simulink model "EngineModel_scaled_27_7_2016_with_new_maps"  (R2021a)
settings: Solver=ode4  StartTime=0.0  StopTime=30  FixedStep=0.2  RelTol=1e-3  EnableMultiTasking=on
values from neighbouring files (symbols this model uses):
  Fanmap_2 = [1 1 1 1 1 1 1 1 1 1 275.724 325.4224 ... (330 elements, 10x3x11)]    [enginemaps2.mat]
  HPCompmap_2 = [1 1 1 1 1 1 1 1 1 1 32.390865 37.6623195 ... (330 elements, 10x3x11)]    [enginemaps2.mat]
  HPTurbinemap_2 = [0.24979968 0.24979968 0.24979968 0.24979968 0.24979968 0.24979968 0.24979968 0.24979968 0.24979968 0.24979968 0.004250667 0.005047667 ... (330 elements, 10x3x11)]    [enginemaps2.mat]
  LPCompmap_2 = [1 1 1 1 1 1 1 1 1 1 34.17260994 40.23277722 ... (330 elements, 10x3x11)]    [enginemaps2.mat]
  LPTurbinemap_2 = [0.665969797 0.665969797 0.665969797 0.665969797 0.665969797 0.665969797 0.665969797 0.665969797 0.00912 0.013173333 0.015706667 0.01672 ... (264 elements, 8x3x11)]    [enginemaps2.mat]
undefined symbols (not defined in the file or in its folder): Adiabatic_compression_fan, Adiabatic_compression_HPC, Adiabatic_compression_LPC, coldnozzle, compression_ram, cond_f2, D, datatables, hotnozzle, HPT1, if_Nth, if_Ntl, if_Z, LPT, performance1, thermo_combustor, turbo
libraries: dspmtrx3 x10, aerolibatmos2 x8, dspsigattribs x3, dspsolvers x2, dspfactors x1
(part 11 of 14)

== system EngineModel_scaled_27_7_2016_with_new_maps/Double spool TFE CF6-50 steady state modeling (BOING 747-200)/Error Due to Vs/Error Due To Dv4/HPC/HPC Map/HPComp Map Lookup Table pressure ratio ==
  Corr Speed Nch : Inport
  zch : Inport  Port=2
  3D HPC map Lookup Table pressure ratio : Lookup_n-D  NumberOfTableDimensions=3  BreakpointsForDimension1=[0.562,0.674,0.787,0.899,1,1.034,1.067,1.124,1.236,1.292]  BreakpointsForDimension2=[1,2,3]  BreakpointsForDimension3=[0,0.1,0.2,0.3,0.4,0.5,0.6,0.7,0.8,0.9,1]  IndexSearchMethod=Linear search  Table=HPCompmap_2  InterpMethod=Cubic spline  ExtrapMethod=Cubic spline  OutDataTypeStr=double  RndMeth=Simplest
      settings: InputPortMap=u0,u1,u2
  Constant1 : Constant
  Display : Display
  HPC Prch : Outport
  wires:
  Constant1/1 -> 3D HPC map Lookup Table pressure ratio/2
  Corr Speed Nch/1 -> 3D HPC map Lookup Table pressure ratio/1
  3D HPC map Lookup Table pressure ratio/1 -> HPC Prch/1, Display/1
  zch/1 -> 3D HPC map Lookup Table pressure ratio/3

== system EngineModel_scaled_27_7_2016_with_new_maps/Double spool TFE CF6-50 steady state modeling (BOING 747-200)/Error Due to Vs/Error Due To Dv4/HPC/HPC Map/If condition Zch ==
  Zchi : Inport
  Demux : Demux  Outputs=1
      settings: DisplayOption=none
  Interpreted MATLAB Function : MATLABFcn  MATLABFcn=if_Z(u(1))  OutputDimensions=1
  Mux : Mux  Inputs=1
      settings: DisplayOption=signals
  Zch : Outport
  wires:
  Zchi/1 -> Mux/1
  Demux/1 -> Zch/1
  Mux/1 -> Interpreted MATLAB Function/1
  Interpreted MATLAB Function/1 -> Demux/1

== system EngineModel_scaled_27_7_2016_with_new_maps/Double spool TFE CF6-50 steady state modeling (BOING 747-200)/Error Due to Vs/Error Due To Dv4/HPT/enthalpy_MAPS/HPT map ==
  Nth : Inport
  TFth : Inport  Port=2
  HPT Map lookup Table (DH/T) : Subsystem
  HPT Map lookup Table Efficency : Subsystem
  (DH/T)th : Outport
  etath : Outport  Port=2
  wires:
  HPT Map lookup Table Efficency/1(HPT Ettath) -> etath/1
  HPT Map lookup Table (DH/T)/1(HPT (DH/T)th) -> (DH/T)th/1
  TFth/1 -> HPT Map lookup Table (DH/T)/2(TFth), HPT Map lookup Table Efficency/2(TFth)
  Nth/1 -> HPT Map lookup Table (DH/T)/1(corr speed Nth), HPT Map lookup Table Efficency/1(corr speed Nth)

== system EngineModel_scaled_27_7_2016_with_new_maps/Double spool TFE CF6-50 steady state modeling (BOING 747-200)/Error Due to Vs/Error Due To Dv4/HPT/enthalpy_MAPS/Nch_Nth ==
  Tt4 : Inport
  Tt2.5 : Inport  Port=2
  Nch : Inport  Port=3
  (To)Ref : Constant  Value=288
  (theta4)d : Constant  Value=1.1018
  Display5 : Display
  Product3 : Product  Inputs=***  SaturateOnIntegerOverflow=on  OutDataTypeStr=Inherit: Same as first input
  Product4 : Product  Inputs=*/  SaturateOnIntegerOverflow=on  OutDataTypeStr=Inherit: Same as first input
  Product6 : Product  Inputs=*/  SaturateOnIntegerOverflow=on  OutDataTypeStr=Inherit: Same as first input
  Product7 : Product  Inputs=*/  SaturateOnIntegerOverflow=on  OutDataTypeStr=Inherit: Same as first input
  Sqrt1 : Sqrt  SaturateOnIntegerOverflow=on
  Sqrt2 : Sqrt  SaturateOnIntegerOverflow=on
  const. : Constant  Value=100
  Nth : Outport
  wires:
  Nch/1 -> Product3/3
  Sqrt2/1 -> Product6/1
  Product6/1 -> Product3/2
  (theta4)d/1 -> Product6/2
  Product4/1 -> Sqrt2/1
  Tt2.5/1 -> Product4/1
  Tt4/1 -> Sqrt1/1
  Product3/1 -> Display5/1, Nth/1
  const./1 -> Product7/1
  Sqrt1/1 -> Product7/2
  (To)Ref/1 -> Product4/2
  Product7/1 -> Product3/1

== system EngineModel_scaled_27_7_2016_with_new_maps/Double spool TFE CF6-50 steady state modeling (BOING 747-200)/Error Due to Vs/Error Due To Dv4/LPC/Adiabatic compression/isentropic compression ==
  Tt13 : Inport
  Prcl : Inport  Port=2
  P13 : Inport  Port=3
  Ht13 : Inport  Port=4
  S13 : Inport  Port=5
  etacl : Inport  Port=6
  Demux : Demux
      settings: DisplayOption=none
  Interpreted MATLAB Function : MATLABFcn  MATLABFcn=Adiabatic_compression_LPC(u(1),u(2),u(3),u(4),u(5),u(6))  OutputDimensions=4
  Mux : Mux  Inputs=6
      settings: DisplayOption=signals
  S25 : Outport
  Tt25 : Outport  Port=2
  Pt25 : Outport  Port=3
  Ht25 : Outport  Port=4
  wires:
  Demux/4 -> Ht25/1
  etacl/1 -> Mux/6
  Demux/3 -> S25/1
  S13/1 -> Mux/5
  Ht13/1 -> Mux/4
  Prcl/1 -> Mux/2
  P13/1 -> Mux/3
  Mux/1 -> Interpreted MATLAB Function/1
  Demux/1 -> Tt25/1
  Interpreted MATLAB Function/1 -> Demux/1
  Demux/2 -> Pt25/1
  Tt13/1 -> Mux/1

== system EngineModel_scaled_27_7_2016_with_new_maps/Double spool TFE CF6-50 steady state modeling (BOING 747-200)/Error Due to Vs/Error Due To Dv4/LPC/LPC Map/If condition Zcl ==
  Zcli : Inport
  Demux : Demux  Outputs=1
      settings: DisplayOption=none
  Interpreted MATLAB Function : MATLABFcn  MATLABFcn=if_Z(u(1))  OutputDimensions=1
  Mux : Mux  Inputs=1
      settings: DisplayOption=signals
  Zcl : Outport
  wires:
  Zcli/1 -> Mux/1
  Demux/1 -> Zcl/1
  Mux/1 -> Interpreted MATLAB Function/1
  Interpreted MATLAB Function/1 -> Demux/1

== system EngineModel_scaled_27_7_2016_with_new_maps/Double spool TFE CF6-50 steady state modeling (BOING 747-200)/Error Due to Vs/Error Due To Dv4/LPC/LPC Map/LPC Map Lookuptable efficiency ==
  corr Speed Ncl : Inport
  Zcl : Inport  Port=2
  3D fanmap Lookup Table : Lookup_n-D  NumberOfTableDimensions=3  BreakpointsForDimension1=[0.3,0.4,0.5,0.6,0.7,0.8,0.9,1.0,1.1,1.2]  BreakpointsForDimension2=[1,2,3]  BreakpointsForDimension3=[0,0.1,0.2,0.3,0.4,0.5,0.6,0.7,0.8,0.9,1]  IndexSearchMethod=Linear search  Table=LPCompmap_2  InterpMethod=Cubic spline  ExtrapMethod=Cubic spline  OutDataTypeStr=double  RndMeth=Simplest
      settings: InputPortMap=u0,u1,u2
  Constant1 : Constant  Value=3
  Display : Display
  etacl : Outport
  wires:
  Zcl/1 -> 3D fanmap Lookup Table/3
  3D fanmap Lookup Table/1 -> Display/1, etacl/1
  Constant1/1 -> 3D fanmap Lookup Table/2
  corr Speed Ncl/1 -> 3D fanmap Lookup Table/1

== system EngineModel_scaled_27_7_2016_with_new_maps/Double spool TFE CF6-50 steady state modeling (BOING 747-200)/Error Due to Vs/Error Due To Dv4/LPC/LPC Map/LPC Map Lookuptable massflow ==
  corr Speed Ncl : Inport
  Zcl : Inport  Port=2
  3D fanmap Lookup Table : Lookup_n-D  NumberOfTableDimensions=3  BreakpointsForDimension1=[0.3,0.4,0.5,0.6,0.7,0.8,0.9,1.0,1.1,1.2]  BreakpointsForDimension2=[1,2,3]  BreakpointsForDimension3=[0,0.1,0.2,0.3,0.4,0.5,0.6,0.7,0.8,0.9,1]  IndexSearchMethod=Linear search  Table=LPCompmap_2  InterpMethod=Cubic spline  ExtrapMethod=Cubic spline  OutDataTypeStr=double  RndMeth=Simplest
      settings: InputPortMap=u0,u1,u2
  Constant1 : Constant  Value=2
  Display : Display
  " MFPcl" : Outport
  wires:
  Zcl/1 -> 3D fanmap Lookup Table/3
  3D fanmap Lookup Table/1 -> Display/1, " MFPcl"/1
  Constant1/1 -> 3D fanmap Lookup Table/2
  corr Speed Ncl/1 -> 3D fanmap Lookup Table/1

== system EngineModel_scaled_27_7_2016_with_new_maps/Double spool TFE CF6-50 steady state modeling (BOING 747-200)/Error Due to Vs/Error Due To Dv4/LPC/LPC Map/LPC Map Lookuptable pressure ratio ==
  corr Speed Ncl : Inport
  Zcl : Inport  Port=2
  3D fanmap Lookup Table : Lookup_n-D  NumberOfTableDimensions=3  BreakpointsForDimension1=[0.3,0.4,0.5,0.6,0.7,0.8,0.9,1.0,1.1,1.2]  BreakpointsForDimension2=[1,2,3]  BreakpointsForDimension3=[0,0.1,0.2,0.3,0.4,0.5,0.6,0.7,0.8,0.9,1]  IndexSearchMethod=Linear search  Table=LPCompmap_2  InterpMethod=Cubic spline  ExtrapMethod=Cubic spline  OutDataTypeStr=double  RndMeth=Simplest
      settings: InputPortMap=u0,u1,u2
  Constant1 : Constant
  Display : Display
  " Prcl" : Outport
  wires:
  corr Speed Ncl/1 -> 3D fanmap Lookup Table/1
  Constant1/1 -> 3D fanmap Lookup Table/2
  3D fanmap Lookup Table/1 -> " Prcl"/1, Display/1
  Zcl/1 -> 3D fanmap Lookup Table/3

== system EngineModel_scaled_27_7_2016_with_new_maps/Double spool TFE CF6-50 steady state modeling (BOING 747-200)/Error Due to Vs/Error Due To Dv4/LPT/enthalpy_MAPS/LPT map ==
  Ntl : Inport
  TFtl : Inport  Port=2
  LPT Map lookup Table (DH/T) : Subsystem
  LPT Map lookup Table Efficency : Subsystem
  (DH/T)tl : Outport
  etatl : Outport  Port=2
  wires:
  LPT Map lookup Table Efficency/1(HPT Ettatl) -> etatl/1
  LPT Map lookup Table (DH/T)/1(LPT (DH/T)tl) -> (DH/T)tl/1
  TFtl/1 -> LPT Map lookup Table (DH/T)/2(TFtl), LPT Map lookup Table Efficency/2(TFtl)
  Ntl/1 -> LPT Map lookup Table (DH/T)/1(corr speed Ntl), LPT Map lookup Table Efficency/1(corr speed Ntl)

== system EngineModel_scaled_27_7_2016_with_new_maps/Double spool TFE CF6-50 steady state modeling (BOING 747-200)/Error Due to Vs/Error Due To Dv4/LPT/enthalpy_MAPS/Nch_Nth ==
  Tt45 : Inport
  Tt2 : Inport  Port=2
  Ncf : Inport  Port=3
  (To)Ref : Constant  Value=288
  (theta2)d : Constant  Value=0.9532186
  Display5 : Display
  Product3 : Product  Inputs=**  SaturateOnIntegerOverflow=on  OutDataTypeStr=Inherit: Same as first input
  Product4 : Product  Inputs=*/  SaturateOnIntegerOverflow=on  OutDataTypeStr=Inherit: Same as first input
  Product6 : Product  Inputs=*/  SaturateOnIntegerOverflow=on  OutDataTypeStr=Inherit: Same as first input
  Product7 : Product  Inputs=*/  SaturateOnIntegerOverflow=on  OutDataTypeStr=Inherit: Same as first input
  Product8 : Product  Inputs=**  SaturateOnIntegerOverflow=on  OutDataTypeStr=Inherit: Same as first input
  Sqrt1 : Sqrt  SaturateOnIntegerOverflow=on
  Sqrt2 : Sqrt  SaturateOnIntegerOverflow=on
  const. : Constant  Value=100
  Ntl : Outport
  wires:
  Sqrt2/1 -> Product6/1
  Product6/1 -> Product8/2
  (theta2)d/1 -> Product6/2
  Product4/1 -> Sqrt2/1
  Tt2/1 -> Product4/1
  Tt45/1 -> Sqrt1/1
  Ncf/1 -> Product3/2
  Product3/1 -> Ntl/1, Display5/1
  const./1 -> Product7/1
  Sqrt1/1 -> Product7/2
  Product7/1 -> Product8/1
  (To)Ref/1 -> Product4/2
  Product8/1 -> Product3/1

== system EngineModel_scaled_27_7_2016_with_new_maps/Double spool TFE CF6-50 steady state modeling (BOING 747-200)/Error Due to Vs/Error Due To Dv4/Ram/If condition PRF/If Action Subsystem ==
  In1 : Inport
  Action Port : ActionPort  ActionPortLabel=if(u1 <1)
  Out1 : Outport
  wires:
  In1/1 -> Out1/1

== system EngineModel_scaled_27_7_2016_with_new_maps/Double spool TFE CF6-50 steady state modeling (BOING 747-200)/Error Due to Vs/Error Due To Dv4/Ram/If condition PRF/If Action Subsystem1 ==
  In1 : Inport
  Action Port : ActionPort  ActionPortLabel=else
  Out1 : Outport
  wires:
  In1/1 -> Out1/1

== system EngineModel_scaled_27_7_2016_with_new_maps/Double spool TFE CF6-50 steady state modeling (BOING 747-200)/Error Due to Vs/Error Due To Dv4/Ram/If condition PRF/If Action Subsystem2 ==
  In1 : Inport
  Action Port : ActionPort  ActionPortLabel=elseif(u1>5)
  Out1 : Outport
  wires:
  In1/1 -> Out1/1

== system EngineModel_scaled_27_7_2016_with_new_maps/Double spool TFE CF6-50 steady state modeling (BOING 747-200)/Error Due to Vs/Error Due To Dv5/Combustor/Thermo_combustor/Combustor thermo ==
  Pt4 : Inport
  Ht4 : Inport  Port=2
  F/A : Inport  Port=3
  Cp3 : Inport  Port=4
  Demux : Demux
      settings: DisplayOption=none
  Interpreted MATLAB Function : MATLABFcn  MATLABFcn=thermo_combustor(u(1),u(2),u(3),u(4))  OutputDimensions=4
  Mux : Mux
      settings: DisplayOption=signals
  Tt4 : Outport
  S4 : Outport  Port=2
  Cp4 : Outport  Port=3
  Mw4 : Outport  Port=4
  wires:
  Mux/1 -> Interpreted MATLAB Function/1
  Interpreted MATLAB Function/1 -> Demux/1
  Ht4/1 -> Mux/2
  Pt4/1 -> Mux/1
  F/A/1 -> Mux/3
  Demux/1 -> Tt4/1
  Demux/2 -> S4/1
  Demux/3 -> Cp4/1
  Demux/4 -> Mw4/1
  Cp3/1 -> Mux/4

== system EngineModel_scaled_27_7_2016_with_new_maps/Double spool TFE CF6-50 steady state modeling (BOING 747-200)/Error Due to Vs/Error Due To Dv5/Combustor/combustor o//p pressure/If Action Subsystem ==
  In1 : Inport
  Action Port : ActionPort  ActionPortLabel=if(u1 > 1)
  Out1 : Outport
  wires:
  In1/1 -> Out1/1

== system EngineModel_scaled_27_7_2016_with_new_maps/Double spool TFE CF6-50 steady state modeling (BOING 747-200)/Error Due to Vs/Error Due To Dv5/Combustor/combustor o//p pressure/If Action Subsystem1 ==
  In1 : Inport
  Action Port : ActionPort  ActionPortLabel=else
  Out1 : Outport
  wires:
  In1/1 -> Out1/1

== system EngineModel_scaled_27_7_2016_with_new_maps/Double spool TFE CF6-50 steady state modeling (BOING 747-200)/Error Due to Vs/Error Due To Dv5/Fan/Adiabatic compression/isentropic compression ==
  Tt2 : Inport
  Pr : Inport  Port=2
  Pt2 : Inport  Port=3
  Ht2 : Inport  Port=4
  S2 : Inport  Port=5
  etaf : Inport  Port=6
  Demux : Demux
      settings: DisplayOption=none
  Interpreted MATLAB Function : MATLABFcn  MATLABFcn=Adiabatic_compression_fan(u(1),u(2),u(3),u(4),u(5),u(6))  OutputDimensions=4
  Mux : Mux  Inputs=6
      settings: DisplayOption=signals
  S13 : Outport
  Tt13 : Outport  Port=2
  Pt13 : Outport  Port=3
  Ht13 : Outport  Port=4
  wires:
  Tt2/1 -> Mux/1
  Demux/2 -> Pt13/1
  Interpreted MATLAB Function/1 -> Demux/1
  Demux/1 -> Tt13/1
  Mux/1 -> Interpreted MATLAB Function/1
  Pt2/1 -> Mux/3
  Pr/1 -> Mux/2
  Ht2/1 -> Mux/4
  S2/1 -> Mux/5
  Demux/3 -> S13/1
  etaf/1 -> Mux/6
  Demux/4 -> Ht13/1

== system EngineModel_scaled_27_7_2016_with_new_maps/Double spool TFE CF6-50 steady state modeling (BOING 747-200)/Error Due to Vs/Error Due To Dv5/Fan/Fan Map/Fan Map Lookuptable mass flow ==
  Ncf : Inport
  Zf : Inport  Port=2
  Constant : Constant  Value=2
  Display : Display
  massflow 3D fanmap Lookup Table : Lookup_n-D  NumberOfTableDimensions=3  BreakpointsForDimension1=[0.3,0.4,0.5,0.6,0.7,0.8,0.9,1.0,1.1,1.2]  BreakpointsForDimension2=[1,2,3]  BreakpointsForDimension3=[0,0.1,0.2,0.3,0.4,0.5,0.6,0.7,0.8,0.9,1]  IndexSearchMethod=Linear search  Table=Fanmap_2  InterpMethod=Cubic spline  ExtrapMethod=Cubic spline  OutDataTypeStr=double  RndMeth=Simplest
      settings: InputPortMap=u0,u1,u2
  Fan MFPf : Outport
  wires:
  massflow 3D fanmap Lookup Table/1 -> Fan MFPf/1, Display/1
  Constant/1 -> massflow 3D fanmap Lookup Table/2
  Ncf/1 -> massflow 3D fanmap Lookup Table/1
  Zf/1 -> massflow 3D fanmap Lookup Table/3

== system EngineModel_scaled_27_7_2016_with_new_maps/Double spool TFE CF6-50 steady state modeling (BOING 747-200)/Error Due to Vs/Error Due To Dv5/Fan/Fan Map/Fan Map Lookuptable efficiency ==
  Ncf : Inport
  Zf : Inport  Port=2
  Constant : Constant  Value=3
  Display : Display
  massflow 3D fanmap Lookup Table : Lookup_n-D  NumberOfTableDimensions=3  BreakpointsForDimension1=[0.3,0.4,0.5,0.6,0.7,0.8,0.9,1.0,1.1,1.2]  BreakpointsForDimension2=[1,2,3]  BreakpointsForDimension3=[0,0.1,0.2,0.3,0.4,0.5,0.6,0.7,0.8,0.9,1]  IndexSearchMethod=Linear search  Table=Fanmap_2  InterpMethod=Cubic spline  ExtrapMethod=Cubic spline  OutDataTypeStr=double  RndMeth=Simplest
      settings: InputPortMap=u0,u1,u2
  Fan etaf : Outport
  wires:
  massflow 3D fanmap Lookup Table/1 -> Fan etaf/1, Display/1
  Constant/1 -> massflow 3D fanmap Lookup Table/2
  Ncf/1 -> massflow 3D fanmap Lookup Table/1
  Zf/1 -> massflow 3D fanmap Lookup Table/3

== system EngineModel_scaled_27_7_2016_with_new_maps/Double spool TFE CF6-50 steady state modeling (BOING 747-200)/Error Due to Vs/Error Due To Dv5/Fan/Fan Map/Fan Map Lookuptable pressure ratio ==
  Ncf : Inport
  Zf : Inport  Port=2
  Constant : Constant
  Display : Display
  massflow 3D fanmap Lookup Table : Lookup_n-D  NumberOfTableDimensions=3  BreakpointsForDimension1=[0.3,0.4,0.5,0.6,0.7,0.8,0.9,1.0,1.1,1.2]  BreakpointsForDimension2=[1,2,3]  BreakpointsForDimension3=[0,0.1,0.2,0.3,0.4,0.5,0.6,0.7,0.8,0.9,1]  IndexSearchMethod=Linear search  Table=Fanmap_2  InterpMethod=Cubic spline  ExtrapMethod=Cubic spline  OutDataTypeStr=double  RndMeth=Simplest
      settings: InputPortMap=u0,u1,u2
  Fan Prf : Outport
  wires:
  Zf/1 -> massflow 3D fanmap Lookup Table/3
  Ncf/1 -> massflow 3D fanmap Lookup Table/1
  Constant/1 -> massflow 3D fanmap Lookup Table/2
  massflow 3D fanmap Lookup Table/1 -> Display/1, Fan Prf/1

== system EngineModel_scaled_27_7_2016_with_new_maps/Double spool TFE CF6-50 steady state modeling (BOING 747-200)/Error Due to Vs/Error Due To Dv5/Fan/Fan Map/If condition Zf ==
  Zfi : Inport
  Demux : Demux  Outputs=1
      settings: DisplayOption=none
  Interpreted MATLAB Function : MATLABFcn  MATLABFcn=if_Z(u(1))  OutputDimensions=1
  Mux : Mux  Inputs=1
      settings: DisplayOption=signals
  Zf : Outport
  wires:
  Interpreted MATLAB Function/1 -> Demux/1
  Mux/1 -> Interpreted MATLAB Function/1
  Demux/1 -> Zf/1
  Zfi/1 -> Mux/1

== system EngineModel_scaled_27_7_2016_with_new_maps/Double spool TFE CF6-50 steady state modeling (BOING 747-200)/Error Due to Vs/Error Due To Dv5/HPC/Adiabatic compression/isentropic compression ==
  Tt25 : Inport
  Prcl : Inport  Port=2
  Pt25 : Inport  Port=3
  Ht25 : Inport  Port=4
  S25 : Inport  Port=5
  etacl : Inport  Port=6
  Demux : Demux  Outputs=5
      settings: DisplayOption=none
  Display : Display
  Interpreted MATLAB Function : MATLABFcn  MATLABFcn=Adiabatic_compression_HPC(u(1),u(2),u(3),u(4),u(5),u(6))  OutputDimensions=5
  Mux : Mux  Inputs=6
      settings: DisplayOption=signals
  Tt3 : Outport
  Pt3 : Outport  Port=2
  S3 : Outport  Port=3
  Ht3 : Outport  Port=4
  Cp3 : Outport  Port=5
  wires:
  Tt25/1 -> Mux/1
  Demux/2 -> Pt3/1
  Interpreted MATLAB Function/1 -> Demux/1
  Demux/1 -> Display/1, Tt3/1
  Mux/1 -> Interpreted MATLAB Function/1
  Pt25/1 -> Mux/3
  Prcl/1 -> Mux/2
  Ht25/1 -> Mux/4
  S25/1 -> Mux/5
  Demux/3 -> S3/1
  etacl/1 -> Mux/6
  Demux/4 -> Ht3/1
  Demux/5 -> Cp3/1

== system EngineModel_scaled_27_7_2016_with_new_maps/Double spool TFE CF6-50 steady state modeling (BOING 747-200)/Error Due to Vs/Error Due To Dv5/HPC/HPC Map/HPComp Map Lookup Table Massflow ==
  Corr Speed Nch : Inport
  zch : Inport  Port=2
  3D HPC map Lookup Table massflow : Lookup_n-D  NumberOfTableDimensions=3  BreakpointsForDimension1=[0.562,0.674,0.787,0.899,1,1.034,1.067,1.124,1.236,1.292]  BreakpointsForDimension2=[1,2,3]  BreakpointsForDimension3=[0,0.1,0.2,0.3,0.4,0.5,0.6,0.7,0.8,0.9,1]  IndexSearchMethod=Linear search  Table=HPCompmap_2  InterpMethod=Cubic spline  ExtrapMethod=Cubic spline  OutDataTypeStr=double  RndMeth=Simplest
      settings: InputPortMap=u0,u1,u2
  Constant1 : Constant  Value=2
  Display : Display
  HPC MFPch : Outport
  wires:
  Constant1/1 -> 3D HPC map Lookup Table massflow/2
  Corr Speed Nch/1 -> 3D HPC map Lookup Table massflow/1
  3D HPC map Lookup Table massflow/1 -> HPC MFPch/1, Display/1
  zch/1 -> 3D HPC map Lookup Table massflow/3

== system EngineModel_scaled_27_7_2016_with_new_maps/Double spool TFE CF6-50 steady state modeling (BOING 747-200)/Error Due to Vs/Error Due To Dv5/HPC/HPC Map/HPComp Map Lookup Table efficiency ==
  Corr Speed Nch : Inport
  zch : Inport  Port=2
  3D HPC map Lookup Table efficiency : Lookup_n-D  NumberOfTableDimensions=3  BreakpointsForDimension1=[0.562,0.674,0.787,0.899,1,1.034,1.067,1.124,1.236,1.292]  BreakpointsForDimension2=[1,2,3]  BreakpointsForDimension3=[0,0.1,0.2,0.3,0.4,0.5,0.6,0.7,0.8,0.9,1]  IndexSearchMethod=Linear search  Table=HPCompmap_2  InterpMethod=Cubic spline  ExtrapMethod=Cubic spline  OutDataTypeStr=double  RndMeth=Simplest
      settings: InputPortMap=u0,u1,u2
  Constant1 : Constant  Value=3
  Display : Display
  HPC etach : Outport
  wires:
  Constant1/1 -> 3D HPC map Lookup Table efficiency/2
  Corr Speed Nch/1 -> 3D HPC map Lookup Table efficiency/1
  3D HPC map Lookup Table efficiency/1 -> HPC etach/1, Display/1
  zch/1 -> 3D HPC map Lookup Table efficiency/3

== system EngineModel_scaled_27_7_2016_with_new_maps/Double spool TFE CF6-50 steady state modeling (BOING 747-200)/Error Due to Vs/Error Due To Dv5/HPC/HPC Map/HPComp Map Lookup Table pressure ratio ==
  Corr Speed Nch : Inport
  zch : Inport  Port=2
  3D HPC map Lookup Table pressure ratio : Lookup_n-D  NumberOfTableDimensions=3  BreakpointsForDimension1=[0.562,0.674,0.787,0.899,1,1.034,1.067,1.124,1.236,1.292]  BreakpointsForDimension2=[1,2,3]  BreakpointsForDimension3=[0,0.1,0.2,0.3,0.4,0.5,0.6,0.7,0.8,0.9,1]  IndexSearchMethod=Linear search  Table=HPCompmap_2  InterpMethod=Cubic spline  ExtrapMethod=Cubic spline  OutDataTypeStr=double  RndMeth=Simplest
      settings: InputPortMap=u0,u1,u2
  Constant1 : Constant
  Display : Display
  HPC Prch : Outport
  wires:
  zch/1 -> 3D HPC map Lookup Table pressure ratio/3
  3D HPC map Lookup Table pressure ratio/1 -> Display/1, HPC Prch/1
  Corr Speed Nch/1 -> 3D HPC map Lookup Table pressure ratio/1
  Constant1/1 -> 3D HPC map Lookup Table pressure ratio/2

== system EngineModel_scaled_27_7_2016_with_new_maps/Double spool TFE CF6-50 steady state modeling (BOING 747-200)/Error Due to Vs/Error Due To Dv5/HPC/HPC Map/If condition Zch ==
  Zchi : Inport
  Demux : Demux  Outputs=1
      settings: DisplayOption=none
  Interpreted MATLAB Function : MATLABFcn  MATLABFcn=if_Z(u(1))  OutputDimensions=1
  Mux : Mux  Inputs=1
      settings: DisplayOption=signals
  Zch : Outport
  wires:
  Interpreted MATLAB Function/1 -> Demux/1
  Mux/1 -> Interpreted MATLAB Function/1
  Demux/1 -> Zch/1
  Zchi/1 -> Mux/1

== system EngineModel_scaled_27_7_2016_with_new_maps/Double spool TFE CF6-50 steady state modeling (BOING 747-200)/Error Due to Vs/Error Due To Dv5/HPT/enthalpy_MAPS/HPT map ==
  Nth : Inport
  TFth : Inport  Port=2
  HPT Map lookup Table (DH/T) : Subsystem
  HPT Map lookup Table Efficency : Subsystem
  (DH/T)th : Outport
  etath : Outport  Port=2
  wires:
  Nth/1 -> HPT Map lookup Table Efficency/1(corr speed Nth), HPT Map lookup Table (DH/T)/1(corr speed Nth)
  TFth/1 -> HPT Map lookup Table Efficency/2(TFth), HPT Map lookup Table (DH/T)/2(TFth)
  HPT Map lookup Table (DH/T)/1(HPT (DH/T)th) -> (DH/T)th/1
  HPT Map lookup Table Efficency/1(HPT Ettath) -> etath/1

== system EngineModel_scaled_27_7_2016_with_new_maps/Double spool TFE CF6-50 steady state modeling (BOING 747-200)/Error Due to Vs/Error Due To Dv5/HPT/enthalpy_MAPS/Nch_Nth ==
  Tt4 : Inport
  Tt2.5 : Inport  Port=2
  Nch : Inport  Port=3
  (To)Ref : Constant  Value=288
  (theta4)d : Constant  Value=1.1018
  Display5 : Display
  Product3 : Product  Inputs=***  SaturateOnIntegerOverflow=on  OutDataTypeStr=Inherit: Same as first input
  Product4 : Product  Inputs=*/  SaturateOnIntegerOverflow=on  OutDataTypeStr=Inherit: Same as first input
  Product6 : Product  Inputs=*/  SaturateOnIntegerOverflow=on  OutDataTypeStr=Inherit: Same as first input
  Product7 : Product  Inputs=*/  SaturateOnIntegerOverflow=on  OutDataTypeStr=Inherit: Same as first input
  Sqrt1 : Sqrt  SaturateOnIntegerOverflow=on
  Sqrt2 : Sqrt  SaturateOnIntegerOverflow=on
  const. : Constant  Value=100
  Nth : Outport
  wires:
  Product7/1 -> Product3/1
  (To)Ref/1 -> Product4/2
  Sqrt1/1 -> Product7/2
  const./1 -> Product7/1
  Product3/1 -> Nth/1, Display5/1
  Tt4/1 -> Sqrt1/1
  Tt2.5/1 -> Product4/1
  Product4/1 -> Sqrt2/1
  (theta4)d/1 -> Product6/2
  Product6/1 -> Product3/2
  Sqrt2/1 -> Product6/1
  Nch/1 -> Product3/3

== system EngineModel_scaled_27_7_2016_with_new_maps/Double spool TFE CF6-50 steady state modeling (BOING 747-200)/Error Due to Vs/Error Due To Dv5/LPC/Adiabatic compression/isentropic compression ==
  Tt13 : Inport
  Prcl : Inport  Port=2
  P13 : Inport  Port=3
  Ht13 : Inport  Port=4
  S13 : Inport  Port=5
  etacl : Inport  Port=6
  Demux : Demux
      settings: DisplayOption=none
  Interpreted MATLAB Function : MATLABFcn  MATLABFcn=Adiabatic_compression_LPC(u(1),u(2),u(3),u(4),u(5),u(6))  OutputDimensions=4
  Mux : Mux  Inputs=6
      settings: DisplayOption=signals
  S25 : Outport
  Tt25 : Outport  Port=2
  Pt25 : Outport  Port=3
  Ht25 : Outport  Port=4
  wires:
  Tt13/1 -> Mux/1
  Demux/2 -> Pt25/1
  Interpreted MATLAB Function/1 -> Demux/1
  Demux/1 -> Tt25/1
  Mux/1 -> Interpreted MATLAB Function/1
  P13/1 -> Mux/3
  Prcl/1 -> Mux/2
  Ht13/1 -> Mux/4
  S13/1 -> Mux/5
  Demux/3 -> S25/1
  etacl/1 -> Mux/6
  Demux/4 -> Ht25/1

== system EngineModel_scaled_27_7_2016_with_new_maps/Double spool TFE CF6-50 steady state modeling (BOING 747-200)/Error Due to Vs/Error Due To Dv5/LPC/LPC Map/If condition Zcl ==
  Zcli : Inport
  Demux : Demux  Outputs=1
      settings: DisplayOption=none
  Interpreted MATLAB Function : MATLABFcn  MATLABFcn=if_Z(u(1))  OutputDimensions=1
  Mux : Mux  Inputs=1
      settings: DisplayOption=signals
  Zcl : Outport
  wires:
  Interpreted MATLAB Function/1 -> Demux/1
  Mux/1 -> Interpreted MATLAB Function/1
  Demux/1 -> Zcl/1
  Zcli/1 -> Mux/1

== system EngineModel_scaled_27_7_2016_with_new_maps/Double spool TFE CF6-50 steady state modeling (BOING 747-200)/Error Due to Vs/Error Due To Dv5/LPC/LPC Map/LPC Map Lookuptable efficiency ==
  corr Speed Ncl : Inport
  Zcl : Inport  Port=2
  3D fanmap Lookup Table : Lookup_n-D  NumberOfTableDimensions=3  BreakpointsForDimension1=[0.3,0.4,0.5,0.6,0.7,0.8,0.9,1.0,1.1,1.2]  BreakpointsForDimension2=[1,2,3]  BreakpointsForDimension3=[0,0.1,0.2,0.3,0.4,0.5,0.6,0.7,0.8,0.9,1]  IndexSearchMethod=Linear search  Table=LPCompmap_2  InterpMethod=Cubic spline  ExtrapMethod=Cubic spline  OutDataTypeStr=double  RndMeth=Simplest
      settings: InputPortMap=u0,u1,u2
  Constant1 : Constant  Value=3
  Display : Display
  etacl : Outport
  wires:
  corr Speed Ncl/1 -> 3D fanmap Lookup Table/1
  Constant1/1 -> 3D fanmap Lookup Table/2
  3D fanmap Lookup Table/1 -> etacl/1, Display/1
  Zcl/1 -> 3D fanmap Lookup Table/3

== system EngineModel_scaled_27_7_2016_with_new_maps/Double spool TFE CF6-50 steady state modeling (BOING 747-200)/Error Due to Vs/Error Due To Dv5/LPC/LPC Map/LPC Map Lookuptable massflow ==
  corr Speed Ncl : Inport
  Zcl : Inport  Port=2
  3D fanmap Lookup Table : Lookup_n-D  NumberOfTableDimensions=3  BreakpointsForDimension1=[0.3,0.4,0.5,0.6,0.7,0.8,0.9,1.0,1.1,1.2]  BreakpointsForDimension2=[1,2,3]  BreakpointsForDimension3=[0,0.1,0.2,0.3,0.4,0.5,0.6,0.7,0.8,0.9,1]  IndexSearchMethod=Linear search  Table=LPCompmap_2  InterpMethod=Cubic spline  ExtrapMethod=Cubic spline  OutDataTypeStr=double  RndMeth=Simplest
      settings: InputPortMap=u0,u1,u2
  Constant1 : Constant  Value=2
  Display : Display
  " MFPcl" : Outport
  wires:
  corr Speed Ncl/1 -> 3D fanmap Lookup Table/1
  Constant1/1 -> 3D fanmap Lookup Table/2
  3D fanmap Lookup Table/1 -> " MFPcl"/1, Display/1
  Zcl/1 -> 3D fanmap Lookup Table/3

== system EngineModel_scaled_27_7_2016_with_new_maps/Double spool TFE CF6-50 steady state modeling (BOING 747-200)/Error Due to Vs/Error Due To Dv5/LPC/LPC Map/LPC Map Lookuptable pressure ratio ==
  corr Speed Ncl : Inport
  Zcl : Inport  Port=2
  3D fanmap Lookup Table : Lookup_n-D  NumberOfTableDimensions=3  BreakpointsForDimension1=[0.3,0.4,0.5,0.6,0.7,0.8,0.9,1.0,1.1,1.2]  BreakpointsForDimension2=[1,2,3]  BreakpointsForDimension3=[0,0.1,0.2,0.3,0.4,0.5,0.6,0.7,0.8,0.9,1]  IndexSearchMethod=Linear search  Table=LPCompmap_2  InterpMethod=Cubic spline  ExtrapMethod=Cubic spline  OutDataTypeStr=double  RndMeth=Simplest
      settings: InputPortMap=u0,u1,u2
  Constant1 : Constant
  Display : Display
  " Prcl" : Outport
  wires:
  Zcl/1 -> 3D fanmap Lookup Table/3
  3D fanmap Lookup Table/1 -> Display/1, " Prcl"/1
  Constant1/1 -> 3D fanmap Lookup Table/2
  corr Speed Ncl/1 -> 3D fanmap Lookup Table/1

== system EngineModel_scaled_27_7_2016_with_new_maps/Double spool TFE CF6-50 steady state modeling (BOING 747-200)/Error Due to Vs/Error Due To Dv5/LPT/enthalpy_MAPS/LPT map ==
  Ntl : Inport
  TFtl : Inport  Port=2
  LPT Map lookup Table (DH/T) : Subsystem
  LPT Map lookup Table Efficency : Subsystem
  (DH/T)tl : Outport
  etatl : Outport  Port=2
  wires:
  Ntl/1 -> LPT Map lookup Table Efficency/1(corr speed Ntl), LPT Map lookup Table (DH/T)/1(corr speed Ntl)
  TFtl/1 -> LPT Map lookup Table Efficency/2(TFtl), LPT Map lookup Table (DH/T)/2(TFtl)
  LPT Map lookup Table (DH/T)/1(LPT (DH/T)tl) -> (DH/T)tl/1
  LPT Map lookup Table Efficency/1(HPT Ettatl) -> etatl/1

== system EngineModel_scaled_27_7_2016_with_new_maps/Double spool TFE CF6-50 steady state modeling (BOING 747-200)/Error Due to Vs/Error Due To Dv5/LPT/enthalpy_MAPS/Nch_Nth ==
  Tt45 : Inport
  Tt2 : Inport  Port=2
  Ncf : Inport  Port=3
  (To)Ref : Constant  Value=288
  (theta2)d : Constant  Value=0.9532186
  Display5 : Display
  Product3 : Product  Inputs=**  SaturateOnIntegerOverflow=on  OutDataTypeStr=Inherit: Same as first input
  Product4 : Product  Inputs=*/  SaturateOnIntegerOverflow=on  OutDataTypeStr=Inherit: Same as first input
  Product6 : Product  Inputs=*/  SaturateOnIntegerOverflow=on  OutDataTypeStr=Inherit: Same as first input
  Product7 : Product  Inputs=*/  SaturateOnIntegerOverflow=on  OutDataTypeStr=Inherit: Same as first input
  Product8 : Product  Inputs=**  SaturateOnIntegerOverflow=on  OutDataTypeStr=Inherit: Same as first input
  Sqrt1 : Sqrt  SaturateOnIntegerOverflow=on
  Sqrt2 : Sqrt  SaturateOnIntegerOverflow=on
  const. : Constant  Value=100
  Ntl : Outport
  wires:
  Product8/1 -> Product3/1
  (To)Ref/1 -> Product4/2
  Product7/1 -> Product8/1
  Sqrt1/1 -> Product7/2
  const./1 -> Product7/1
  Product3/1 -> Display5/1, Ntl/1
  Ncf/1 -> Product3/2
  Tt45/1 -> Sqrt1/1
  Tt2/1 -> Product4/1
  Product4/1 -> Sqrt2/1
  (theta2)d/1 -> Product6/2
  Product6/1 -> Product8/2
  Sqrt2/1 -> Product6/1

== system EngineModel_scaled_27_7_2016_with_new_maps/Double spool TFE CF6-50 steady state modeling (BOING 747-200)/Error Due to Vs/Error Due To Dv5/Ram/If condition PRF/If Action Subsystem ==
  In1 : Inport
  Action Port : ActionPort  ActionPortLabel=if(u1 <1)
  Out1 : Outport
  wires:
  In1/1 -> Out1/1

== system EngineModel_scaled_27_7_2016_with_new_maps/Double spool TFE CF6-50 steady state modeling (BOING 747-200)/Error Due to Vs/Error Due To Dv5/Ram/If condition PRF/If Action Subsystem1 ==
  In1 : Inport
  Action Port : ActionPort  ActionPortLabel=else
  Out1 : Outport
  wires:
  In1/1 -> Out1/1

== system EngineModel_scaled_27_7_2016_with_new_maps/Double spool TFE CF6-50 steady state modeling (BOING 747-200)/Error Due to Vs/Error Due To Dv5/Ram/If condition PRF/If Action Subsystem2 ==
  In1 : Inport
  Action Port : ActionPort  ActionPortLabel=elseif(u1>5)
  Out1 : Outport
  wires:
  In1/1 -> Out1/1

== system EngineModel_scaled_27_7_2016_with_new_maps/Double spool TFE CF6-50 steady state modeling (BOING 747-200)/Error Due to Vs/Error Due To Dv6/Combustor/Thermo_combustor/Combustor thermo ==
  Pt4 : Inport
  Ht4 : Inport  Port=2
  F/A : Inport  Port=3
  Cp3 : Inport  Port=4
  Demux : Demux
      settings: DisplayOption=none
  Interpreted MATLAB Function : MATLABFcn  MATLABFcn=thermo_combustor(u(1),u(2),u(3),u(4))  OutputDimensions=4
  Mux : Mux
      settings: DisplayOption=signals
  Tt4 : Outport
  S4 : Outport  Port=2
  Cp4 : Outport  Port=3
  Mw4 : Outport  Port=4
  wires:
  Cp3/1 -> Mux/4
  Demux/4 -> Mw4/1
  Demux/3 -> Cp4/1
  Demux/2 -> S4/1
  Demux/1 -> Tt4/1
  F/A/1 -> Mux/3
  Pt4/1 -> Mux/1
  Ht4/1 -> Mux/2
  Interpreted MATLAB Function/1 -> Demux/1
  Mux/1 -> Interpreted MATLAB Function/1

== system EngineModel_scaled_27_7_2016_with_new_maps/Double spool TFE CF6-50 steady state modeling (BOING 747-200)/Error Due to Vs/Error Due To Dv6/Combustor/combustor o//p pressure/If Action Subsystem ==
  In1 : Inport
  Action Port : ActionPort  ActionPortLabel=if(u1 > 1)
  Out1 : Outport
  wires:
  In1/1 -> Out1/1

== system EngineModel_scaled_27_7_2016_with_new_maps/Double spool TFE CF6-50 steady state modeling (BOING 747-200)/Error Due to Vs/Error Due To Dv6/Combustor/combustor o//p pressure/If Action Subsystem1 ==
  In1 : Inport
  Action Port : ActionPort  ActionPortLabel=else
  Out1 : Outport
  wires:
  In1/1 -> Out1/1

== system EngineModel_scaled_27_7_2016_with_new_maps/Double spool TFE CF6-50 steady state modeling (BOING 747-200)/Error Due to Vs/Error Due To Dv6/Fan/Adiabatic compression/isentropic compression ==
  Tt2 : Inport
  Pr : Inport  Port=2
  Pt2 : Inport  Port=3
  Ht2 : Inport  Port=4
  S2 : Inport  Port=5
  etaf : Inport  Port=6
  Demux : Demux
      settings: DisplayOption=none
  Interpreted MATLAB Function : MATLABFcn  MATLABFcn=Adiabatic_compression_fan(u(1),u(2),u(3),u(4),u(5),u(6))  OutputDimensions=4
  Mux : Mux  Inputs=6
      settings: DisplayOption=signals
  S13 : Outport
  Tt13 : Outport  Port=2
  Pt13 : Outport  Port=3
  Ht13 : Outport  Port=4
  wires:
  Demux/4 -> Ht13/1
  etaf/1 -> Mux/6
  Demux/3 -> S13/1
  S2/1 -> Mux/5
  Ht2/1 -> Mux/4
  Pr/1 -> Mux/2
  Pt2/1 -> Mux/3
  Mux/1 -> Interpreted MATLAB Function/1
  Demux/1 -> Tt13/1
  Interpreted MATLAB Function/1 -> Demux/1
  Demux/2 -> Pt13/1
  Tt2/1 -> Mux/1

== system EngineModel_scaled_27_7_2016_with_new_maps/Double spool TFE CF6-50 steady state modeling (BOING 747-200)/Error Due to Vs/Error Due To Dv6/Fan/Fan Map/Fan Map Lookuptable mass flow ==
  Ncf : Inport
  Zf : Inport  Port=2
  Constant : Constant  Value=2
  Display : Display
  massflow 3D fanmap Lookup Table : Lookup_n-D  NumberOfTableDimensions=3  BreakpointsForDimension1=[0.3,0.4,0.5,0.6,0.7,0.8,0.9,1.0,1.1,1.2]  BreakpointsForDimension2=[1,2,3]  BreakpointsForDimension3=[0,0.1,0.2,0.3,0.4,0.5,0.6,0.7,0.8,0.9,1]  IndexSearchMethod=Linear search  Table=Fanmap_2  InterpMethod=Cubic spline  ExtrapMethod=Cubic spline  OutDataTypeStr=double  RndMeth=Simplest
      settings: InputPortMap=u0,u1,u2
  Fan MFPf : Outport
  wires:
  Zf/1 -> massflow 3D fanmap Lookup Table/3
  Ncf/1 -> massflow 3D fanmap Lookup Table/1
  Constant/1 -> massflow 3D fanmap Lookup Table/2
  massflow 3D fanmap Lookup Table/1 -> Display/1, Fan MFPf/1

== system EngineModel_scaled_27_7_2016_with_new_maps/Double spool TFE CF6-50 steady state modeling (BOING 747-200)/Error Due to Vs/Error Due To Dv6/Fan/Fan Map/Fan Map Lookuptable efficiency ==
  Ncf : Inport
  Zf : Inport  Port=2
  Constant : Constant  Value=3
  Display : Display
  massflow 3D fanmap Lookup Table : Lookup_n-D  NumberOfTableDimensions=3  BreakpointsForDimension1=[0.3,0.4,0.5,0.6,0.7,0.8,0.9,1.0,1.1,1.2]  BreakpointsForDimension2=[1,2,3]  BreakpointsForDimension3=[0,0.1,0.2,0.3,0.4,0.5,0.6,0.7,0.8,0.9,1]  IndexSearchMethod=Linear search  Table=Fanmap_2  InterpMethod=Cubic spline  ExtrapMethod=Cubic spline  OutDataTypeStr=double  RndMeth=Simplest
      settings: InputPortMap=u0,u1,u2
  Fan etaf : Outport
  wires:
  Zf/1 -> massflow 3D fanmap Lookup Table/3
  Ncf/1 -> massflow 3D fanmap Lookup Table/1
  Constant/1 -> massflow 3D fanmap Lookup Table/2
  massflow 3D fanmap Lookup Table/1 -> Display/1, Fan etaf/1

== system EngineModel_scaled_27_7_2016_with_new_maps/Double spool TFE CF6-50 steady state modeling (BOING 747-200)/Error Due to Vs/Error Due To Dv6/Fan/Fan Map/Fan Map Lookuptable pressure ratio ==
  Ncf : Inport
  Zf : Inport  Port=2
  Constant : Constant
  Display : Display
  massflow 3D fanmap Lookup Table : Lookup_n-D  NumberOfTableDimensions=3  BreakpointsForDimension1=[0.3,0.4,0.5,0.6,0.7,0.8,0.9,1.0,1.1,1.2]  BreakpointsForDimension2=[1,2,3]  BreakpointsForDimension3=[0,0.1,0.2,0.3,0.4,0.5,0.6,0.7,0.8,0.9,1]  IndexSearchMethod=Linear search  Table=Fanmap_2  InterpMethod=Cubic spline  ExtrapMethod=Cubic spline  OutDataTypeStr=double  RndMeth=Simplest
      settings: InputPortMap=u0,u1,u2
  Fan Prf : Outport
  wires:
  massflow 3D fanmap Lookup Table/1 -> Fan Prf/1, Display/1
  Constant/1 -> massflow 3D fanmap Lookup Table/2
  Ncf/1 -> massflow 3D fanmap Lookup Table/1
  Zf/1 -> massflow 3D fanmap Lookup Table/3

== system EngineModel_scaled_27_7_2016_with_new_maps/Double spool TFE CF6-50 steady state modeling (BOING 747-200)/Error Due to Vs/Error Due To Dv6/Fan/Fan Map/If condition Zf ==
  Zfi : Inport
  Demux : Demux  Outputs=1
      settings: DisplayOption=none
  Interpreted MATLAB Function : MATLABFcn  MATLABFcn=if_Z(u(1))  OutputDimensions=1
  Mux : Mux  Inputs=1
      settings: DisplayOption=signals
  Zf : Outport
  wires:
  Zfi/1 -> Mux/1
  Demux/1 -> Zf/1
  Mux/1 -> Interpreted MATLAB Function/1
  Interpreted MATLAB Function/1 -> Demux/1

== system EngineModel_scaled_27_7_2016_with_new_maps/Double spool TFE CF6-50 steady state modeling (BOING 747-200)/Error Due to Vs/Error Due To Dv6/HPC/Adiabatic compression/isentropic compression ==
  Tt25 : Inport
  Prcl : Inport  Port=2
  Pt25 : Inport  Port=3
  Ht25 : Inport  Port=4
  S25 : Inport  Port=5
  etacl : Inport  Port=6
  Demux : Demux  Outputs=5
      settings: DisplayOption=none
  Display : Display
  Interpreted MATLAB Function : MATLABFcn  MATLABFcn=Adiabatic_compression_HPC(u(1),u(2),u(3),u(4),u(5),u(6))  OutputDimensions=5
  Mux : Mux  Inputs=6
      settings: DisplayOption=signals
  Tt3 : Outport
  Pt3 : Outport  Port=2
  S3 : Outport  Port=3
  Ht3 : Outport  Port=4
  Cp3 : Outport  Port=5
  wires:
  Demux/5 -> Cp3/1
  Demux/4 -> Ht3/1
  etacl/1 -> Mux/6
  Demux/3 -> S3/1
  S25/1 -> Mux/5
  Ht25/1 -> Mux/4
  Prcl/1 -> Mux/2
  Pt25/1 -> Mux/3
  Mux/1 -> Interpreted MATLAB Function/1
  Demux/1 -> Tt3/1, Display/1
  Interpreted MATLAB Function/1 -> Demux/1
  Demux/2 -> Pt3/1
  Tt25/1 -> Mux/1

== system EngineModel_scaled_27_7_2016_with_new_maps/Double spool TFE CF6-50 steady state modeling (BOING 747-200)/Error Due to Vs/Error Due To Dv6/HPC/HPC Map/HPComp Map Lookup Table Massflow ==
  Corr Speed Nch : Inport
  zch : Inport  Port=2
  3D HPC map Lookup Table massflow : Lookup_n-D  NumberOfTableDimensions=3  BreakpointsForDimension1=[0.562,0.674,0.787,0.899,1,1.034,1.067,1.124,1.236,1.292]  BreakpointsForDimension2=[1,2,3]  BreakpointsForDimension3=[0,0.1,0.2,0.3,0.4,0.5,0.6,0.7,0.8,0.9,1]  IndexSearchMethod=Linear search  Table=HPCompmap_2  InterpMethod=Cubic spline  ExtrapMethod=Cubic spline  OutDataTypeStr=double  RndMeth=Simplest
      settings: InputPortMap=u0,u1,u2
  Constant1 : Constant  Value=2
  Display : Display
  HPC MFPch : Outport
  wires:
  zch/1 -> 3D HPC map Lookup Table massflow/3
  3D HPC map Lookup Table massflow/1 -> Display/1, HPC MFPch/1
  Corr Speed Nch/1 -> 3D HPC map Lookup Table massflow/1
  Constant1/1 -> 3D HPC map Lookup Table massflow/2

== system EngineModel_scaled_27_7_2016_with_new_maps/Double spool TFE CF6-50 steady state modeling (BOING 747-200)/Error Due to Vs/Error Due To Dv6/HPC/HPC Map/HPComp Map Lookup Table efficiency ==
  Corr Speed Nch : Inport
  zch : Inport  Port=2
  3D HPC map Lookup Table efficiency : Lookup_n-D  NumberOfTableDimensions=3  BreakpointsForDimension1=[0.562,0.674,0.787,0.899,1,1.034,1.067,1.124,1.236,1.292]  BreakpointsForDimension2=[1,2,3]  BreakpointsForDimension3=[0,0.1,0.2,0.3,0.4,0.5,0.6,0.7,0.8,0.9,1]  IndexSearchMethod=Linear search  Table=HPCompmap_2  InterpMethod=Cubic spline  ExtrapMethod=Cubic spline  OutDataTypeStr=double  RndMeth=Simplest
      settings: InputPortMap=u0,u1,u2
  Constant1 : Constant  Value=3
  Display : Display
  HPC etach : Outport
  wires:
  zch/1 -> 3D HPC map Lookup Table efficiency/3
  3D HPC map Lookup Table efficiency/1 -> Display/1, HPC etach/1
  Corr Speed Nch/1 -> 3D HPC map Lookup Table efficiency/1
  Constant1/1 -> 3D HPC map Lookup Table efficiency/2

== system EngineModel_scaled_27_7_2016_with_new_maps/Double spool TFE CF6-50 steady state modeling (BOING 747-200)/Error Due to Vs/Error Due To Dv6/HPC/HPC Map/HPComp Map Lookup Table pressure ratio ==
  Corr Speed Nch : Inport
  zch : Inport  Port=2
  3D HPC map Lookup Table pressure ratio : Lookup_n-D  NumberOfTableDimensions=3  BreakpointsForDimension1=[0.562,0.674,0.787,0.899,1,1.034,1.067,1.124,1.236,1.292]  BreakpointsForDimension2=[1,2,3]  BreakpointsForDimension3=[0,0.1,0.2,0.3,0.4,0.5,0.6,0.7,0.8,0.9,1]  IndexSearchMethod=Linear search  Table=HPCompmap_2  InterpMethod=Cubic spline  ExtrapMethod=Cubic spline  OutDataTypeStr=double  RndMeth=Simplest
      settings: InputPortMap=u0,u1,u2
  Constant1 : Constant
  Display : Display
  HPC Prch : Outport
  wires:
  Constant1/1 -> 3D HPC map Lookup Table pressure ratio/2
  Corr Speed Nch/1 -> 3D HPC map Lookup Table pressure ratio/1
  3D HPC map Lookup Table pressure ratio/1 -> HPC Prch/1, Display/1
  zch/1 -> 3D HPC map Lookup Table pressure ratio/3

== system EngineModel_scaled_27_7_2016_with_new_maps/Double spool TFE CF6-50 steady state modeling (BOING 747-200)/Error Due to Vs/Error Due To Dv6/HPC/HPC Map/If condition Zch ==
  Zchi : Inport
  Demux : Demux  Outputs=1
      settings: DisplayOption=none
  Interpreted MATLAB Function : MATLABFcn  MATLABFcn=if_Z(u(1))  OutputDimensions=1
  Mux : Mux  Inputs=1
      settings: DisplayOption=signals
  Zch : Outport
  wires:
  Zchi/1 -> Mux/1
  Demux/1 -> Zch/1
  Mux/1 -> Interpreted MATLAB Function/1
  Interpreted MATLAB Function/1 -> Demux/1

== system EngineModel_scaled_27_7_2016_with_new_maps/Double spool TFE CF6-50 steady state modeling (BOING 747-200)/Error Due to Vs/Error Due To Dv6/HPT/enthalpy_MAPS/HPT map ==
  Nth : Inport
  TFth : Inport  Port=2
  HPT Map lookup Table (DH/T) : Subsystem
  HPT Map lookup Table Efficency : Subsystem
  (DH/T)th : Outport
  etath : Outport  Port=2
  wires:
  HPT Map lookup Table Efficency/1(HPT Ettath) -> etath/1
  HPT Map lookup Table (DH/T)/1(HPT (DH/T)th) -> (DH/T)th/1
  TFth/1 -> HPT Map lookup Table (DH/T)/2(TFth), HPT Map lookup Table Efficency/2(TFth)
  Nth/1 -> HPT Map lookup Table (DH/T)/1(corr speed Nth), HPT Map lookup Table Efficency/1(corr speed Nth)

== system EngineModel_scaled_27_7_2016_with_new_maps/Double spool TFE CF6-50 steady state modeling (BOING 747-200)/Error Due to Vs/Error Due To Dv6/HPT/enthalpy_MAPS/Nch_Nth ==
  Tt4 : Inport
  Tt2.5 : Inport  Port=2
  Nch : Inport  Port=3
  (To)Ref : Constant  Value=288
  (theta4)d : Constant  Value=1.1018
  Display5 : Display
  Product3 : Product  Inputs=***  SaturateOnIntegerOverflow=on  OutDataTypeStr=Inherit: Same as first input
  Product4 : Product  Inputs=*/  SaturateOnIntegerOverflow=on  OutDataTypeStr=Inherit: Same as first input
  Product6 : Product  Inputs=*/  SaturateOnIntegerOverflow=on  OutDataTypeStr=Inherit: Same as first input
  Product7 : Product  Inputs=*/  SaturateOnIntegerOverflow=on  OutDataTypeStr=Inherit: Same as first input
  Sqrt1 : Sqrt  SaturateOnIntegerOverflow=on
  Sqrt2 : Sqrt  SaturateOnIntegerOverflow=on
  const. : Constant  Value=100
  Nth : Outport
  wires:
  Nch/1 -> Product3/3
  Sqrt2/1 -> Product6/1
  Product6/1 -> Product3/2
  (theta4)d/1 -> Product6/2
  Product4/1 -> Sqrt2/1
  Tt2.5/1 -> Product4/1
  Tt4/1 -> Sqrt1/1
  Product3/1 -> Display5/1, Nth/1
  const./1 -> Product7/1
  Sqrt1/1 -> Product7/2
  (To)Ref/1 -> Product4/2
  Product7/1 -> Product3/1

== system EngineModel_scaled_27_7_2016_with_new_maps/Double spool TFE CF6-50 steady state modeling (BOING 747-200)/Error Due to Vs/Error Due To Dv6/LPC/Adiabatic compression/isentropic compression ==
  Tt13 : Inport
  Prcl : Inport  Port=2
  P13 : Inport  Port=3
  Ht13 : Inport  Port=4
  S13 : Inport  Port=5
  etacl : Inport  Port=6
  Demux : Demux
      settings: DisplayOption=none
  Interpreted MATLAB Function : MATLABFcn  MATLABFcn=Adiabatic_compression_LPC(u(1),u(2),u(3),u(4),u(5),u(6))  OutputDimensions=4
  Mux : Mux  Inputs=6
      settings: DisplayOption=signals
  S25 : Outport
  Tt25 : Outport  Port=2
  Pt25 : Outport  Port=3
  Ht25 : Outport  Port=4
  wires:
  Demux/4 -> Ht25/1
  etacl/1 -> Mux/6
  Demux/3 -> S25/1
  S13/1 -> Mux/5
  Ht13/1 -> Mux/4
  Prcl/1 -> Mux/2
  P13/1 -> Mux/3
  Mux/1 -> Interpreted MATLAB Function/1
  Demux/1 -> Tt25/1
  Interpreted MATLAB Function/1 -> Demux/1
  Demux/2 -> Pt25/1
  Tt13/1 -> Mux/1

== system EngineModel_scaled_27_7_2016_with_new_maps/Double spool TFE CF6-50 steady state modeling (BOING 747-200)/Error Due to Vs/Error Due To Dv6/LPC/LPC Map/If condition Zcl ==
  Zcli : Inport
  Demux : Demux  Outputs=1
      settings: DisplayOption=none
  Interpreted MATLAB Function : MATLABFcn  MATLABFcn=if_Z(u(1))  OutputDimensions=1
  Mux : Mux  Inputs=1
      settings: DisplayOption=signals
  Zcl : Outport
  wires:
  Zcli/1 -> Mux/1
  Demux/1 -> Zcl/1
  Mux/1 -> Interpreted MATLAB Function/1
  Interpreted MATLAB Function/1 -> Demux/1

== system EngineModel_scaled_27_7_2016_with_new_maps/Double spool TFE CF6-50 steady state modeling (BOING 747-200)/Error Due to Vs/Error Due To Dv6/LPC/LPC Map/LPC Map Lookuptable efficiency ==
  corr Speed Ncl : Inport
  Zcl : Inport  Port=2
  3D fanmap Lookup Table : Lookup_n-D  NumberOfTableDimensions=3  BreakpointsForDimension1=[0.3,0.4,0.5,0.6,0.7,0.8,0.9,1.0,1.1,1.2]  BreakpointsForDimension2=[1,2,3]  BreakpointsForDimension3=[0,0.1,0.2,0.3,0.4,0.5,0.6,0.7,0.8,0.9,1]  IndexSearchMethod=Linear search  Table=LPCompmap_2  InterpMethod=Cubic spline  ExtrapMethod=Cubic spline  OutDataTypeStr=double  RndMeth=Simplest
      settings: InputPortMap=u0,u1,u2
  Constant1 : Constant  Value=3
  Display : Display
  etacl : Outport
  wires:
  Zcl/1 -> 3D fanmap Lookup Table/3
  3D fanmap Lookup Table/1 -> Display/1, etacl/1
  Constant1/1 -> 3D fanmap Lookup Table/2
  corr Speed Ncl/1 -> 3D fanmap Lookup Table/1

== system EngineModel_scaled_27_7_2016_with_new_maps/Double spool TFE CF6-50 steady state modeling (BOING 747-200)/Error Due to Vs/Error Due To Dv6/LPC/LPC Map/LPC Map Lookuptable massflow ==
  corr Speed Ncl : Inport
  Zcl : Inport  Port=2
  3D fanmap Lookup Table : Lookup_n-D  NumberOfTableDimensions=3  BreakpointsForDimension1=[0.3,0.4,0.5,0.6,0.7,0.8,0.9,1.0,1.1,1.2]  BreakpointsForDimension2=[1,2,3]  BreakpointsForDimension3=[0,0.1,0.2,0.3,0.4,0.5,0.6,0.7,0.8,0.9,1]  IndexSearchMethod=Linear search  Table=LPCompmap_2  InterpMethod=Cubic spline  ExtrapMethod=Cubic spline  OutDataTypeStr=double  RndMeth=Simplest
      settings: InputPortMap=u0,u1,u2
  Constant1 : Constant  Value=2
  Display : Display
  " MFPcl" : Outport
  wires:
  Zcl/1 -> 3D fanmap Lookup Table/3
  3D fanmap Lookup Table/1 -> Display/1, " MFPcl"/1
  Constant1/1 -> 3D fanmap Lookup Table/2
  corr Speed Ncl/1 -> 3D fanmap Lookup Table/1

== system EngineModel_scaled_27_7_2016_with_new_maps/Double spool TFE CF6-50 steady state modeling (BOING 747-200)/Error Due to Vs/Error Due To Dv6/LPC/LPC Map/LPC Map Lookuptable pressure ratio ==
  corr Speed Ncl : Inport
  Zcl : Inport  Port=2
  3D fanmap Lookup Table : Lookup_n-D  NumberOfTableDimensions=3  BreakpointsForDimension1=[0.3,0.4,0.5,0.6,0.7,0.8,0.9,1.0,1.1,1.2]  BreakpointsForDimension2=[1,2,3]  BreakpointsForDimension3=[0,0.1,0.2,0.3,0.4,0.5,0.6,0.7,0.8,0.9,1]  IndexSearchMethod=Linear search  Table=LPCompmap_2  InterpMethod=Cubic spline  ExtrapMethod=Cubic spline  OutDataTypeStr=double  RndMeth=Simplest
      settings: InputPortMap=u0,u1,u2
  Constant1 : Constant
  Display : Display
  " Prcl" : Outport
  wires:
  corr Speed Ncl/1 -> 3D fanmap Lookup Table/1
  Constant1/1 -> 3D fanmap Lookup Table/2
  3D fanmap Lookup Table/1 -> " Prcl"/1, Display/1
  Zcl/1 -> 3D fanmap Lookup Table/3

== system EngineModel_scaled_27_7_2016_with_new_maps/Double spool TFE CF6-50 steady state modeling (BOING 747-200)/Error Due to Vs/Error Due To Dv6/LPT/enthalpy_MAPS/LPT map ==
  Ntl : Inport
  TFtl : Inport  Port=2
  LPT Map lookup Table (DH/T) : Subsystem
  LPT Map lookup Table Efficency : Subsystem
  (DH/T)tl : Outport
  etatl : Outport  Port=2
  wires:
  LPT Map lookup Table Efficency/1(HPT Ettatl) -> etatl/1
  LPT Map lookup Table (DH/T)/1(LPT (DH/T)tl) -> (DH/T)tl/1
  TFtl/1 -> LPT Map lookup Table (DH/T)/2(TFtl), LPT Map lookup Table Efficency/2(TFtl)
  Ntl/1 -> LPT Map lookup Table (DH/T)/1(corr speed Ntl), LPT Map lookup Table Efficency/1(corr speed Ntl)

== system EngineModel_scaled_27_7_2016_with_new_maps/Double spool TFE CF6-50 steady state modeling (BOING 747-200)/Error Due to Vs/Error Due To Dv6/LPT/enthalpy_MAPS/Nch_Nth ==
  Tt45 : Inport
  Tt2 : Inport  Port=2
  Ncf : Inport  Port=3
  (To)Ref : Constant  Value=288
  (theta2)d : Constant  Value=0.9532186
  Display5 : Display
  Product3 : Product  Inputs=**  SaturateOnIntegerOverflow=on  OutDataTypeStr=Inherit: Same as first input
  Product4 : Product  Inputs=*/  SaturateOnIntegerOverflow=on  OutDataTypeStr=Inherit: Same as first input
  Product6 : Product  Inputs=*/  SaturateOnIntegerOverflow=on  OutDataTypeStr=Inherit: Same as first input
  Product7 : Product  Inputs=*/  SaturateOnIntegerOverflow=on  OutDataTypeStr=Inherit: Same as first input
  Product8 : Product  Inputs=**  SaturateOnIntegerOverflow=on  OutDataTypeStr=Inherit: Same as first input
  Sqrt1 : Sqrt  SaturateOnIntegerOverflow=on
  Sqrt2 : Sqrt  SaturateOnIntegerOverflow=on
  const. : Constant  Value=100
  Ntl : Outport
  wires:
  Sqrt2/1 -> Product6/1
  Product6/1 -> Product8/2
  (theta2)d/1 -> Product6/2
  Product4/1 -> Sqrt2/1
  Tt2/1 -> Product4/1
  Tt45/1 -> Sqrt1/1
  Ncf/1 -> Product3/2
  Product3/1 -> Ntl/1, Display5/1
  const./1 -> Product7/1
  Sqrt1/1 -> Product7/2
  Product7/1 -> Product8/1
  (To)Ref/1 -> Product4/2
  Product8/1 -> Product3/1
